simulink model "simulinkTemp"  (R2023b)
settings: Solver=VariableStepAuto  StartTime=0.0  StopTime=450  RelTol=1e-3
libraries: cstblocks x3
settings Model: Creator=daas0  LastModifiedBy=daas0

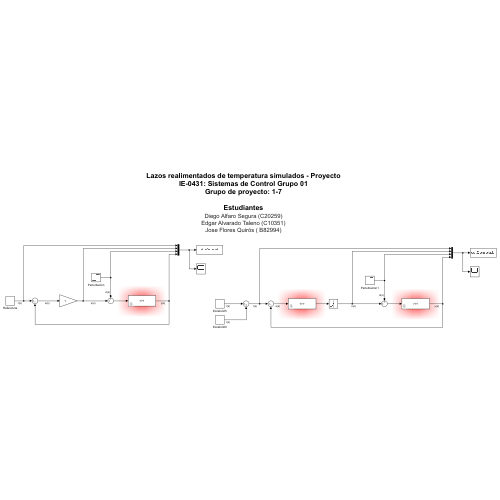
[thumbnail: Simulink's stored preview of the top-level diagram]
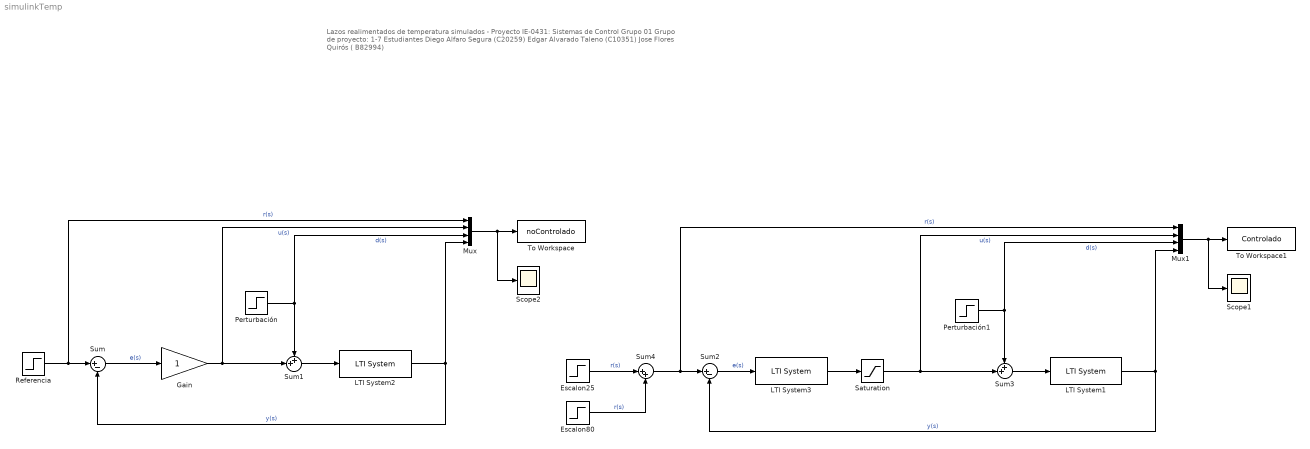
== system simulinkTemp ==
  note: Lazos realimentados de temperatura simulados - Proyecto
      | IE-0431: Sistemas de Control Grupo 01
      | Grupo de proyecto: 1-7
      |
      | Estudiantes
      | Diego Alfaro Segura (C20259)
      | Edgar Alvarado Taleno (C10351)
      | Jose Flores Quirós ( B82994)
  Escalon25 : Step  Time=0  After=25  SampleTime=0
  Escalon80 : Step  Time=150  After=55  SampleTime=0
  Gain : Gain
  LTI System1 : cstblocks/LTI System  sys=temp_G  IC=[]  PadeOrder=0
  LTI System2 : cstblocks/LTI System  sys=temp_G  IC=[]  PadeOrder=0
  LTI System3 : cstblocks/LTI System  sys=controladorPID  IC=[]  PadeOrder=0
  Mux : Mux
  Mux1 : Mux
  Perturbación : Step  Time=200  After=20  SampleTime=0
  Perturbación1 : Step  Time=300  After=20  SampleTime=0
  Referencia : Step  Time=0  After=20  SampleTime=0
  Saturation : Saturate  UpperLimit=100
  Scope1 : Scope
  Scope2 : Scope
  Sum : Sum  Inputs=|+-
  Sum1 : Sum  Inputs=++|
  Sum2 : Sum  Inputs=|+-
  Sum3 : Sum  Inputs=++|
  Sum4 : Sum  Inputs=|++
  To Workspace : ToWorkspace  VariableName=noControlado  SaveFormat=Timeseries  SampleTime=-1
  To Workspace1 : ToWorkspace  VariableName=Controlado  SaveFormat=Timeseries  SampleTime=-1
  wires:
  LTI System2/1 -> Mux/4, Sum/2  "y(s)"
  Sum/1 -> Gain/1  "e(s)"
  Referencia/1 -> Mux/1, Sum/1  "r(s)"
  Gain/1 -> Mux/2, Sum1/2  "u(s)"
  Sum1/1 -> LTI System2/1
  Perturbación/1 -> Sum1/1, Mux/3  "d(s)"
  Mux/1 -> Scope2/1, To Workspace/1
  Mux1/1 -> Scope1/1, To Workspace1/1
  Perturbación1/1 -> Sum3/1, Mux1/3  "d(s)"
  Sum4/1 -> Mux1/1, Sum2/1  "r(s)"
  LTI System1/1 -> Mux1/4, Sum2/2  "y(s)"
  Sum3/1 -> LTI System1/1
  Escalon25/1 -> Sum4/1  "r(s)"
  Escalon80/1 -> Sum4/2  "r(s)"
  Saturation/1 -> Mux1/2, Sum3/2  "u(s)"
  LTI System3/1 -> Saturation/1
  Sum2/1 -> LTI System3/1  "e(s)"
